simulink model "AutomatedParkingValet1"  (R2018a)
settings: Solver=ode3  StartTime=0.0  StopTime=Inf  FixedStep=0.01  MinStep=1e-3  RelTol=5e-3
PreLoadFcn:
  | costmap = helperSLCreateCostmap();
  | routeData= load('routePlan.mat');
  | routePlan= routeData.routePlan;
  | startPose = routePlan.StartPose(1, :);
  | helperSLCreateUtilityBus;
StopFcn:
  | clear helperSLBehaviorPlanning ...
  | helperSLFeedbackController ...
  | helperSLMotionPlanning ...
  | helperSLGenerateSmoothPath ...
  | helperSLGenerateSpeedProfile ...
  | helperSLVisualizePath;
libraries: autolibshared x1
CloseFcn:
  | clear elemsPath ...
  | elemsPlannerConfig ...
  | elemsSpeedConfig ...
  | elemsSpline ...
  | pathBus ...
  | plannerConfigBus ...
  | speedConfigBus ...
  | splineDataBus ...
  | startPose ...
  | costmap ...
  | routeData ...
  | routePlan;
settings Model: Creator=The MathWorks, Inc.  LastModifiedBy=jdrjk
settings SolverCC: ZeroCrossAlgorithm=Adaptive  DecoupledContinuousIntegration=on  MinimalZcImpactIntegration=on
settings DataIOCC: SaveOutput=off  SignalLogging=off  DSMLogging=off  SaveTime=off

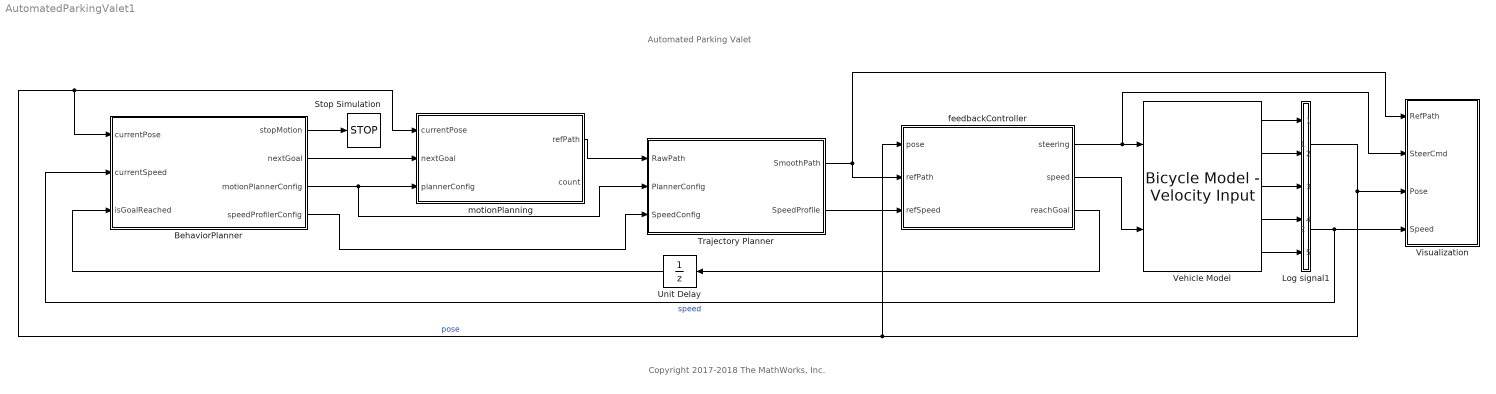
== system AutomatedParkingValet1 ==
  note: Copyright 2017-2018 The MathWorks, Inc.
  note: Automated Parking Valet
  BehaviorPlanner : MATLAB Function  TreatAsAtomicUnit=on  mask{Costmap=costmap, RoutePlan=routePlan, StartSpeed=0}
      mask prompts: Costmap "Vehicle costmap:"; RoutePlan "Route plan:"; StartSpeed "Initial vehicle speed  [m/s]:"
      mask init:
      | validateattributes(Costmap, {'vehicleCostmap'}, {'scalar'});
      | validateattributes(RoutePlan, {'table'}, {'ncols', 3});
      | validateattributes(StartSpeed, {'double'}, {'scalar','nonnegative'})
      | 
      | routePlanStruct   = table2struct(RoutePlan);
      | startPose         = routePlanStruct(1).StartPose;
      | 
      | varagout          = helperSLCreateUtilityStruct(Costmap);
      | vehicleDimsStruct = varagout{1};
      | costmapStruct     = varagout{2};
  Log signal1 : Subsystem
  Stop Simulation : Stop
  Trajectory Planner : Subsystem  mask{Costmap=costmap}
      mask prompts: Costmap "Vehicle costmap:"
      mask init:
      | validateattributes(Costmap, {'vehicleCostmap'}, {'scalar'});
      | 
      | varagout          = helperSLCreateUtilityStruct(Costmap);
      | vehicleDimsStruct = varagout{1};
      | costmapStruct     = varagout{2};
      mask DialogControl DescTextVar Prompt: Generate a smooth path and a speed profile along the path.
      mask Display:
      | disp(['Trajectory' char(10) 'Generator']);
      | port_label('input',1,'RefPath');
      | port_label('input',2,'PlannerConfig');
      | port_label('input',3,'SpeedConfig');
      | 
      | port_label('output',1,'SmoothPath');
      | port_label('output',2,'RefSpeed');
  Unit Delay : UnitDelay  SampleTime=-1
  Vehicle Model : autolibshared/Bicycle Model - Velocity Input  trackMode=Single (bicycle)  inputMode=External longitudinal forces  frontSteerMode=on  rearSteerMode=off  windMode=off  muMode=off  extFMode=off  extMMode=off  aMode=3  NF=2  NR=2  m=2000  a=costmap.VehicleDimensions.Wheelbase/2  b=costmap.VehicleDimensions.Wheelbase/2  h=costmap.VehicleDimensions.Height  X_o=startPose(1) + cosd(startPose(3)) * costmap.VehicleDimensions.Wheelbase/2  xdot_o=0  CalphaMode=off  sigmaMode=on  w=[1.4,1.4]  Cy_f=12e3  Cy_r=11e3  sigma_f=.1  sigma_r=.1  alpha_f_brk=[-.1 .1]  Cy_f_data=[-9e3 9e3]  alpha_r_brk=[-.1 .1]  Cy_r_data=[-9e3 9e3]  Y_o=startPose(2) + sind(startPose(3)) * costmap.VehicleDimensions.Wheelbase/2  ydot_o=0  Izz=4000  psi_o=0  r_o=0  Af=2  Cd=.3  Cl=.1  Cpm=.1  beta_w=[0:0.01:0.3]  Cs=[0:0.03:0.9]  Cym=[0:0.01:0.3]  Pabs=101325  Tair=273  g=9.81  mu=1  xdot_tol=.01  Fznom=5000  Fxtire_sat=1e6  Fytire_sat=1e6
      settings: SourceProductName=Powertrain Blockset  SourceProductBaseCode=PW
  Visualization : Subsystem  mask{Costmap=costmap}
      mask prompts: Costmap "Vehicle costmap:"
      mask init:
      | validateattributes(Costmap, {'vehicleCostmap'}, {'scalar'});
      | 
      | varagout          = helperSLCreateUtilityStruct(Costmap);
      | vehicleDimsStruct = varagout{1};
      | costmapStruct     = varagout{2};
      mask DialogControl DescTextVar Prompt: Visualize simulation results.
  feedbackController : MATLAB Function  TreatAsAtomicUnit=on  mask{VehicleDims=costmap.VehicleDimensions, StartSpeed=0, StartSteer=0}
      mask prompts: VehicleDims "Vehicle dimensions:"; StartSpeed "Initial vehicle speed [m/s]:"; StartSteer "Initial steering angle [deg]:"
      mask init:
      | validateattributes(VehicleDims, {'vehicleDimensions'}, {'scalar'});
      | 
      | varagout          = helperSLCreateUtilityStruct(VehicleDims);
      | vehicleDimsStruct = varagout{1};
  motionPlanning : MATLAB Function  TreatAsAtomicUnit=on  mask{Costmap=costmap, MinIterations=1000, ConnectionDistance=10, MinTurningRadius=20, XStart=startPose(1), YStart=startPose(2), ThetaStart=startPose(3)}
      mask prompts: Costmap "Vehicle costmap:"; MinIterations "Minimum iteration:"; ConnectionDistance "Connection distance [m]:"; MinTurningRadius "Minimum turning radius [m]:"; XStart "X positon [m]:"; YStart "Y position [m]:"; ThetaStart "Heading angle [deg]:"
      mask init:
      | validateattributes(Costmap, {'vehicleCostmap'}, {'scalar'});
      | 
      | startPose         = [XStart, YStart, ThetaStart];
      | 
      | varagout          = helperSLCreateUtilityStruct(Costmap);
      | vehicleDimsStruct = varagout{1};
      | costmapStruct     = varagout{2};
  wires:
  Log signal1/1(pose) -> feedbackController/1(pose), motionPlanning/1(currentPose), BehaviorPlanner/1(currentPose), Visualization/3(Pose)  "pose"
  Trajectory Planner/1(SmoothPath) -> feedbackController/2(refPath), Visualization/1(RefPath)
  Trajectory Planner/2(SpeedProfile) -> feedbackController/3(refSpeed)
  Log signal1/2(speed) -> BehaviorPlanner/2(currentSpeed), Visualization/4(Speed)  "speed"
  Unit Delay/1 -> BehaviorPlanner/3(isGoalReached)
  BehaviorPlanner/2(nextGoal) -> motionPlanning/2(nextGoal)
  motionPlanning/1(refPath) -> Trajectory Planner/1(RawPath)
  feedbackController/1(steering) -> Visualization/2(SteerCmd), Vehicle Model/1
  feedbackController/2(speed) -> Vehicle Model/2
  Vehicle Model/1 -> Log signal1/1(In1)
  Vehicle Model/2 -> Log signal1/2(In2)
  Vehicle Model/3 -> Log signal1/3(In3)
  Vehicle Model/4 -> Log signal1/4(In4)
  Vehicle Model/5 -> Log signal1/5(In5)
  BehaviorPlanner/3(motionPlannerConfig) -> motionPlanning/3(plannerConfig), Trajectory Planner/2(PlannerConfig)
  BehaviorPlanner/4(speedProfilerConfig) -> Trajectory Planner/3(SpeedConfig)
  BehaviorPlanner/1(stopMotion) -> Stop Simulation/1
  feedbackController/3(reachGoal) -> Unit Delay/1

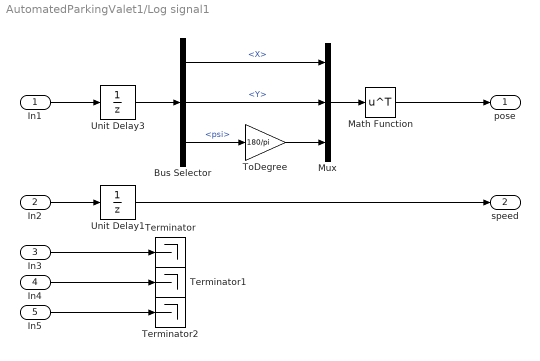
== system AutomatedParkingValet1/Log signal1 ==
  In1 : Inport
  In2 : Inport  Port=2
  In3 : Inport  Port=3
  In4 : Inport  Port=4
  In5 : Inport  Port=5
  Bus Selector : BusSelector  OutputSignals=InertFrm.RearAxl.Disp.X,InertFrm.RearAxl.Disp.Y,InertFrm.Cg.Ang.psi
  Math Function : Math  Operator=transpose  SaturateOnIntegerOverflow=on
  Mux : Mux  Inputs=3
  Terminator : Terminator
  Terminator1 : Terminator
  Terminator2 : Terminator
  ToDegree : Gain  Gain=180/pi
  Unit Delay1 : UnitDelay  SampleTime=-1
  Unit Delay3 : UnitDelay  SampleTime=-1
  pose : Outport
  speed : Outport  Port=2
  wires:
  In4/1 -> Terminator1/1
  Bus Selector/3 -> ToDegree/1  "<psi>"
  In5/1 -> Terminator2/1
  In1/1 -> Unit Delay3/1
  In3/1 -> Terminator/1
  Unit Delay3/1 -> Bus Selector/1
  In2/1 -> Unit Delay1/1
  Unit Delay1/1 -> speed/1
  Mux/1 -> Math Function/1
  Bus Selector/1 -> Mux/1  "<X>"
  Bus Selector/2 -> Mux/2  "<Y>"
  ToDegree/1 -> Mux/3
  Math Function/1 -> pose/1

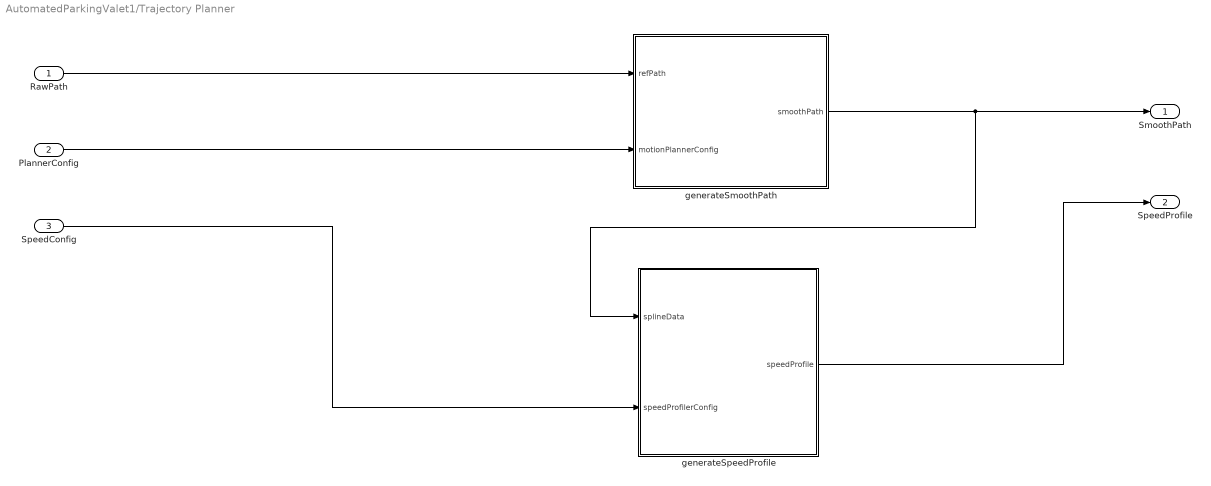
== system AutomatedParkingValet1/Trajectory Planner ==
  RawPath : Inport
  PlannerConfig : Inport  Port=2
  SpeedConfig : Inport  Port=3
  generateSmoothPath : MATLAB Function  TreatAsAtomicUnit=on
  generateSpeedProfile : MATLAB Function  TreatAsAtomicUnit=on
  SmoothPath : Outport
  SpeedProfile : Outport  Port=2
  wires:
  generateSmoothPath/1(smoothPath) -> SmoothPath/1, generateSpeedProfile/1(splineData)
  RawPath/1 -> generateSmoothPath/1(refPath)
  generateSpeedProfile/1(speedProfile) -> SpeedProfile/1
  PlannerConfig/1 -> generateSmoothPath/2(motionPlannerConfig)
  SpeedConfig/1 -> generateSpeedProfile/2(speedProfilerConfig)

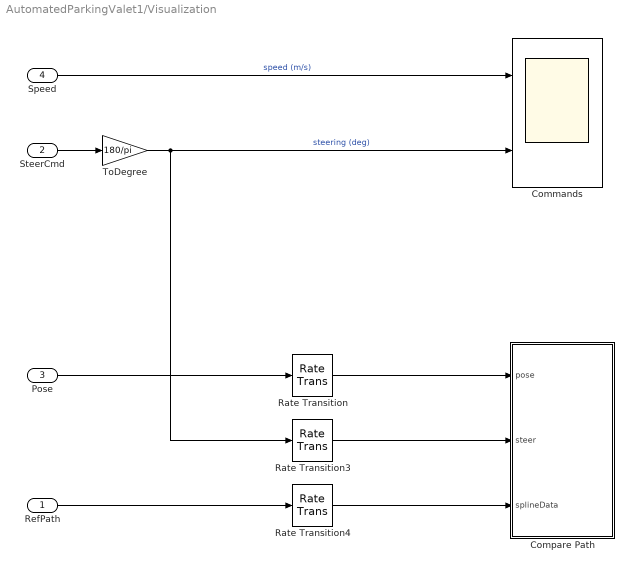
== system AutomatedParkingValet1/Visualization ==
  RefPath : Inport
  SteerCmd : Inport  Port=2
  Pose : Inport  Port=3
  Speed : Inport  Port=4
  Commands : Scope  NumInputPorts=2
  Compare Path : MATLAB Function  TreatAsAtomicUnit=on
  Rate Transition : RateTransition  OutPortSampleTime=0.2
  Rate Transition3 : RateTransition  OutPortSampleTime=0.2
  Rate Transition4 : RateTransition  OutPortSampleTime=0.2
  ToDegree : Gain  Gain=180/pi
  wires:
  Rate Transition/1 -> Compare Path/1(pose)
  Rate Transition4/1 -> Compare Path/3(splineData)
  Rate Transition3/1 -> Compare Path/2(steer)
  Speed/1 -> Commands/1  "speed (m/s)"
  RefPath/1 -> Rate Transition4/1
  SteerCmd/1 -> ToDegree/1
  Pose/1 -> Rate Transition/1
  ToDegree/1 -> Commands/2, Rate Transition3/1  "steering (deg)"

== matlab function AutomatedParkingValet1/motionPlanning ==
  data: refPath output Bus: pathBus; currentPose input; nextGoal input; startPose parameter; plannerConfig input Bus: plannerConfigBus; costmapStruct parameter; vehicleDimsStruct parameter; ConnectionDistance parameter; MinTurningRadius parameter; MinIterations parameter; count output
function [refPath, count] = motionPlanning(currentPose, nextGoal, startPose, ...
    plannerConfig, costmapStruct, vehicleDimsStruct, ...
    ConnectionDistance, MinTurningRadius, MinIterations)

%motionPlanning plan a feasible path.

coder.extrinsic('helperSLMotionPlanning');

refPath = helperSLMotionPlanning(costmapStruct, vehicleDimsStruct, ...
    currentPose, nextGoal, plannerConfig, startPose, ...
    MinIterations, ConnectionDistance, MinTurningRadius);

persistent counter;
if(isempty(counter))
    counter = 0;
end
counter = counter + 1;
count = counter;

== matlab function AutomatedParkingValet1/Trajectory Planner/generateSpeedProfile ==
  data: splineData input Bus: splineDataBus; speedProfile output; speedProfilerConfig input Bus: speedConfigBus
function speedProfile = generateSpeedProfile(splineData, speedProfilerConfig)

%generateSpeedProfile generate a speed profile along the reference path.

coder.extrinsic('helperSLGenerateSpeedProfile');

speedProfile = coder.nullcopy(zeros(size(splineData.x ,1), 1));

speedProfile = helperSLGenerateSpeedProfile(splineData, speedProfilerConfig);

== matlab function AutomatedParkingValet1/Trajectory Planner/generateSmoothPath ==
  data: refPath input; motionPlannerConfig input; smoothPath output Bus: splineDataBus; costmapStruct parameter
function smoothPath = generateSmoothPath(refPath, motionPlannerConfig, costmapStruct)

%generateSmoothPath generate a smooth path.

coder.extrinsic('helperSLGenerateSmoothPath');

smoothPath = helperSLGenerateSmoothPath(refPath, motionPlannerConfig, costmapStruct);

== matlab function AutomatedParkingValet1/feedbackController ==
  data: steering output size=1; speed output size=1; pose input; reachGoal output boolean size=1; refPath input; refSpeed input; vehicleDimsStruct parameter; StartSteer parameter; StartSpeed parameter
function [steering, speed, reachGoal] = feedbackController(...
    pose, refPath, refSpeed, vehicleDimsStruct, StartSteer, StartSpeed)

%feedbackController compute control commands to drive the vehicle.

coder.extrinsic('helperSLFeedbackController');

speed     = coder.nullcopy(0);
steering  = coder.nullcopy(0);
reachGoal = coder.nullcopy(logical(0));  %#ok<*LOGL,*NASGU>

[speed, steering, reachGoal] = helperSLFeedbackController(...
    pose, vehicleDimsStruct, refPath, refSpeed, StartSteer, StartSpeed);

steering = deg2rad(steering);

== matlab function AutomatedParkingValet1/Visualization/Compare Path ==
  data: pose input; steer input; splineData input; costmapStruct parameter; vehicleDimsStruct parameter
function visualizePath(pose, steer, splineData, costmapStruct, vehicleDimsStruct)

%visualizePath Display simulation results.

coder.extrinsic('helperSLVisualizePath');

helperSLVisualizePath(pose, steer, splineData, costmapStruct, vehicleDimsStruct)

== matlab function AutomatedParkingValet1/BehaviorPlanner ==
  data: stopMotion output; nextGoal output double size=[1 3]; motionPlannerConfig output Bus: plannerConfigBus; speedProfilerConfig output Bus: speedConfigBus; routePlanStruct parameter; currentPose input; currentSpeed input; isGoalReached input; costmapStruct parameter; vehicleDimsStruct parameter; startPose parameter; StartSpeed parameter
function [stopMotion, nextGoal, motionPlannerConfig, speedProfilerConfig] = ...
    behaviorPlanning(routePlanStruct, currentPose, currentSpeed, isGoalReached, ...
    costmapStruct, vehicleDimsStruct, startPose, StartSpeed)

%behaviorPlanning generate navigation tasks and configurations for the 
%   Motion Planner block and the Trajectory Generator block.

coder.extrinsic('helperSLBehaviorPlanning');

nextGoal     = coder.nullcopy(zeros(1, 3)); %#ok<*NASGU>
stopMotion   = coder.nullcopy(logical(0));  %#ok<*LOGL>

[nextGoal, motionPlannerConfig, speedProfilerConfig, stopMotion] = ...
    helperSLBehaviorPlanning(costmapStruct, vehicleDimsStruct, ...
    routePlanStruct, currentPose, currentSpeed, isGoalReached, ...
    startPose, StartSpeed);

end
